simulink model "models_for_drawings"  (R2017a)
settings: Solver=VariableStepAuto  StartTime=0.0  StopTime=10.0  RelTol=1e-3
undefined symbols (not defined in the file or in its folder): Kp, L_s
libraries: elec_lib x2, fl_lib x1
settings Model: Creator=mac_daino  LastModifiedBy=mac_daino

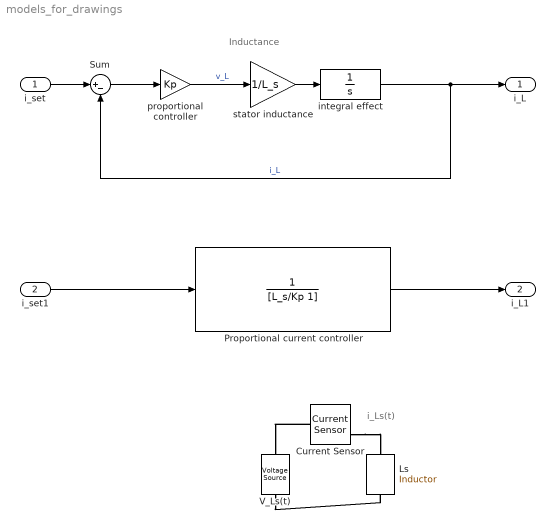
== system models_for_drawings ==
  note: i_Ls(t)
  note: Inductance
  i_set : Inport
  i_set1 : Inport  Port=2
  Current Sensor : fl_lib/Electrical/Electrical Sensors/Current Sensor
  Ls : elec_lib/Passive Devices/Inductor  l=L H  L_tol=20  enable_L_tol=0  tol_distribution=1  nSigma=4  r=0 Ohm  g=1e-9 1/Ohm  enable_operating_limits=0  operating_limit_action=2  max_working_current=1 A  power_rating=1 W  enable_faults=0  fault_action=1  lambdaPercent=50  k_faulted=0.9999  turnsShort=0  openCct=0  groundShort=0  groundShortG=0 1/Ohm  tau_fault=1e-3 s  enable_temporal_fault=0  t_fault=1 s  enable_behavioral_fault=0  max_permissible_voltage=100 V  n_fail_on_voltage=1  max_permissible_current=1 A  t_fail_on_current=1 s  i_L_specify=off  i_L_priority=High  i_L=0 A  i_L_nominal_specify=off  i_L_nominal_unit=A  i_L_nominal_value=1
      settings: SourceProductName=Simscape Electronics  SourceProductBaseCode=SN
  Proportional current controller : TransferFcn  Denominator=[L_s/Kp 1]
  Sum : Sum  Inputs=|+-
  V_Ls(t) : elec_lib/Sources/Voltage Source  dc_voltage=V_Ls V  ac_voltage=0 V  ac_shift=0 rad  ac_frequency=60 Hz  noise_mode=0  PSD=0 V^2/Hz  repeatability=1  auto_seed=3510290603  user_seed=0  sample_time=1e-3 s  i_specify=off  i_priority=None  i=0 A  i_nominal_specify=off  i_nominal_unit=A  i_nominal_value=1  v_specify=off  v_priority=None  v=0 V  v_nominal_specify=off  v_nominal_unit=V  v_nominal_value=1
      settings: SourceProductName=Simscape Electronics  SourceProductBaseCode=SN
  integral effect : Integrator
  proportional controller : Gain  Gain=Kp
  stator inductance : Gain  Gain=1/L_s
  i_L : Outport
  i_L1 : Outport  Port=2
  wires:
  stator inductance/1 -> integral effect/1
  proportional controller/1 -> stator inductance/1  "v_L"
  Sum/1 -> proportional controller/1
  integral effect/1 -> i_L/1, Sum/2  "i_L"
  i_set/1 -> Sum/1
  Proportional current controller/1 -> i_L1/1
  i_set1/1 -> Proportional current controller/1
  connections:
  V_Ls(t)/RConn1 -- Ls/RConn1
  Current Sensor/RConn2 -- Ls/LConn1
  Current Sensor/LConn1 -- V_Ls(t)/LConn1
